simulink model "FullBalekaRaibert"  (R2025a)
settings: Solver=VariableStepAuto  StartTime=0.0  StopTime=20  RelTol=1e-3
libraries: aru_toolbox x4, simulink x2
settings Model: Creator=Gavin  LastModifiedBy=Gavin
settings ExplorerConfigSet: InternalSimMechanicsExplorerSettings=|
  | <ExplorerConfiguration>
  | 
  |   <canonicalview>default</canonicalview>
  | 
  |   <TilePanel>
  |     <TileInfo>
  |       <Tiles Columns="1" Count="1" Height="832" Rows="1" Width="1462">
  |         <Row Weight="1"/>
  |         <Column Weight="1"/>
  |         <Tile Height="1" Width="1" X="0" Y="0"/>
  |       </Tiles>
  |     </TileInfo>
  |     <SceneInfo>
  |       <SceneViewer>
  |         <IsThisViewStd>
  |           <IsStandardView>off</IsStandardView>
  |           <StandardViewName>Front</StandardViewName>
  |         </IsThisViewStd>
  |         <BGColor>
  |           <R>1</R>
  |           <G>1</G>
  |           <B>1</B>
  |           <A>1</A>
  |         </BGColor>
  |         <Camera>
  |           <DoPerspective>off</DoPerspective>
  |           <Position>
  |             <X>5.3584715991237664</X>
  |             <Y>-23.628300699422176</Y>
  |             <Z>4.8241020067654929</Z>
  |           </Position>
  |           <Center>
  |             <X>-0.00083063994179468563</X>
  |             <Y>-0.0051618537568766925</Y>
  |             <Z>0.24669244118891392</Z>
  |           </Center>
  |           <Up>
  |             <X>-0.22205533792545343</X>
  |             <Y>0.13668780175983591</Y>
  |             <Z>0.9654055478133925</Z>
  |           </Up>
  |           <XLim>2.6471256395411848</XLim>
  |           <YLim>2.6471256395411848</YLim>
  |           <ViewLimDist>0.01</ViewLimDist>
  |         </Camera>
  |       </SceneViewer>
  |     </SceneInfo>
  |   </TilePanel>
  | 
  |   <MechEditorPanel>
  |     <GfxPanelCameraMap/>
  |     <Cameras>
  |       <Camera>
  |         <Id>Camera1</Id>
  |         <Value>
  |           <Name>FollowBot</Name>
  |           <NativeCamera>
  |             <PositionTrackingFeature>Subsystem.Half_Baleka_Simscape_WIP.Planarising_Boom.Center_to_CameraUp.F</PositionTrackingFeature>
  |             <CenterTrackingFeature>Subsystem.Half_Baleka_Simscape_WIP.Planarising_Boom.Center_to_Camera.B</CenterTrackingFeature>
  |             <UpVectorTrackingFeature>Subsystem.Half_Baleka_Simscape_WIP.Planarising_Boom.Center_to_Camera.B</UpVectorTrackingFeature>
  |             <CenterTrackingOrigin>on</CenterTrackingOrigin>
  |             <UpVectorTrackingDirection>+Y</UpVectorTrackingDirection>
  |           </NativeCamera>
  |         </Value>
  |       </Camera>
  |     </Cameras>
  |     <VideoCreator>
  |       <IncludeTiles>All</IncludeTiles>
  |       <IncludeTime>on</IncludeTime>
  |       <IncludeWorldFrame>off</IncludeWorldFrame>
  |       <PlaybackSpeedRatio>1</PlaybackSpeedRatio>
  |       <FrameRate>30</FrameRate>
  |       <FrameSize>auto</FrameSize>
  |       <VideoFormat>MotionJPEGAVI</VideoFormat>
  |     </VideoCreator>
  |   </MechEditorPanel>
  | 
  |   <PlaybackSettings>
  |     <PlaybackSpeedFactor>1</PlaybackSpeedFactor>
  |   </PlaybackSettings>
  | 
  | </ExplorerConfiguration>

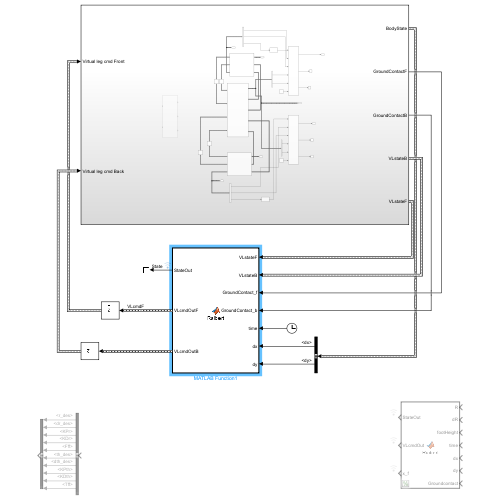
[thumbnail: Simulink's stored preview of the top-level diagram]
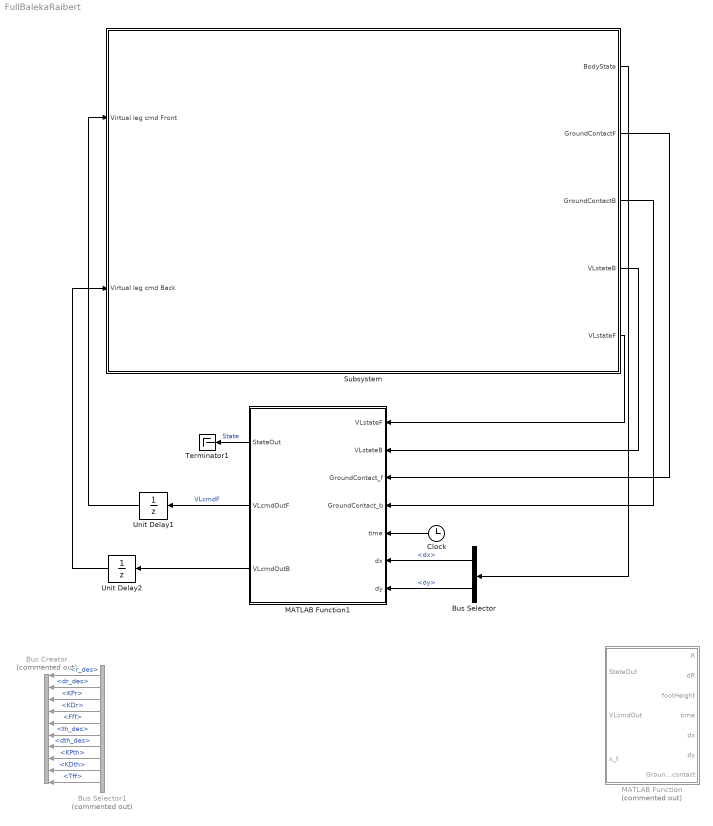
== system FullBalekaRaibert ==
  Bus Creator : BusCreator  Commented=on  Inputs=10  OutDataTypeStr=Bus: VLcmd  NonVirtualBus=on
      settings: InheritFromInputs=off
  Bus Selector : BusSelector  OutputSignals=dx,dy
  Bus Selector1 : BusSelector  Commented=on  OutputSignals=r_des,dr_des,KPr,KDr,Fff,th_des,dth_des,KPth,KDth,Tff
  Clock : Clock
  MATLAB Function : MATLAB Function  Commented=on  TreatAsAtomicUnit=on
  MATLAB Function1 : MATLAB Function  TreatAsAtomicUnit=on
  Subsystem : Subsystem
  Terminator1 : Terminator
  Unit Delay1 : UnitDelay  SampleTime=-1  HasFrameUpgradeWarning=on
  Unit Delay2 : UnitDelay  SampleTime=-1  HasFrameUpgradeWarning=on
  wires:
  MATLAB Function1/1(StateOut) -> Terminator1/1  "State"
  Clock/1 -> MATLAB Function1/5(time)
  Bus Selector/1 -> MATLAB Function1/6(dx)  "<dx>"
  Bus Selector/2 -> MATLAB Function1/7(dy)  "<dy>"
  Bus Selector1/8 -> Bus Creator/8  "<KPth>"
  Bus Selector1/2 -> Bus Creator/2  "<dr_des>"
  Bus Selector1/4 -> Bus Creator/4  "<KDr>"
  Bus Selector1/7 -> Bus Creator/7  "<dth_des>"
  Bus Selector1/5 -> Bus Creator/5  "<Fff>"
  Bus Selector1/6 -> Bus Creator/6  "<th_des>"
  Bus Selector1/3 -> Bus Creator/3  "<KPr>"
  Bus Selector1/10 -> Bus Creator/10  "<Tff>"
  Bus Selector1/9 -> Bus Creator/9  "<KDth>"
  Bus Selector1/1 -> Bus Creator/1  "<r_des>"
  MATLAB Function1/2(VLcmdOutF) -> Unit Delay1/1  "VLcmdF"
  Unit Delay1/1 -> Subsystem/1(Virtual leg cmd Front)
  MATLAB Function1/3(VLcmdOutB) -> Unit Delay2/1
  Unit Delay2/1 -> Subsystem/2(Virtual leg cmd Back)
  Subsystem/1(BodyState) -> Bus Selector/1
  Subsystem/4(VLstateB) -> MATLAB Function1/2(VLstateB)
  Subsystem/3(GroundContactB) -> MATLAB Function1/4(GroundContact_b)
  Subsystem/2(GroundContactF) -> MATLAB Function1/3(GroundContact_f)
  Subsystem/5(VLstateF) -> MATLAB Function1/1(VLstateF)

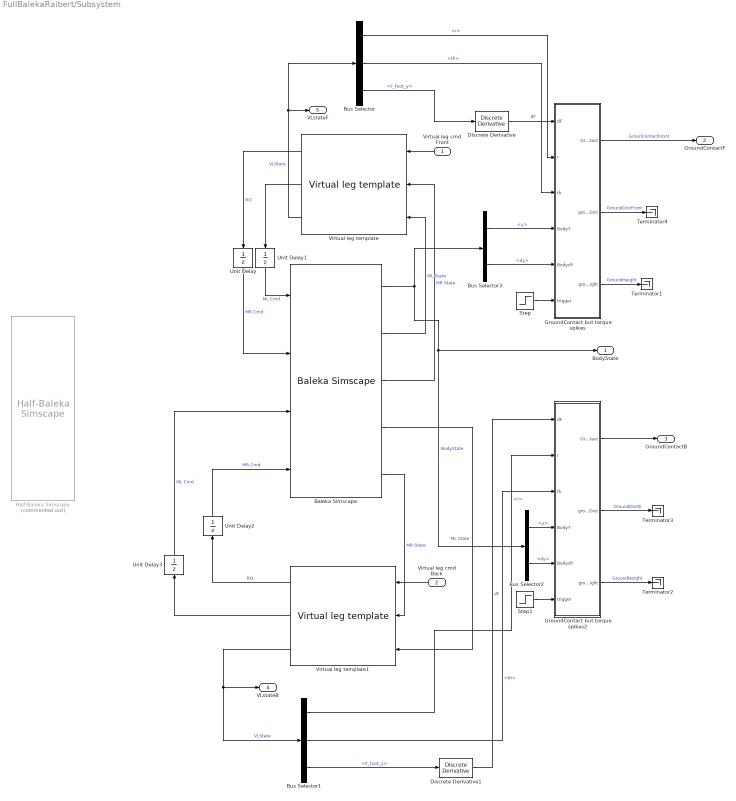
== system FullBalekaRaibert/Subsystem ==
  Virtual leg cmd Front : Inport  OutDataTypeStr=Bus: VLcmd
  Virtual leg cmd Back : Inport  Port=2  OutDataTypeStr=Bus: VLcmd
  Baleka Simscape : aru_toolbox/Baleka 2.5/Baleka Simscape  communication_rate=1000  GravityBool=on  mu_s=1  mu_k=0.9  foot_k=1e5  foot_d=1e4  y_start=0.25  StartingMode=Crouched  LOffset=3*pi/2  ROffset=-pi/2
      settings: SourceProductName=ARU Toolbox
  Bus Selector : BusSelector  OutputSignals=r,th,F_foot_y
  Bus Selector1 : BusSelector  OutputSignals=r,th,F_foot_y
  Bus Selector2 : BusSelector  OutputSignals=y,dy
  Bus Selector3 : BusSelector  OutputSignals=y,dy
  Discrete Derivative : simulink/Discrete/Discrete Derivative  gainval=1.0  ICPrevScaledInput=0.0  OutMin=[]  OutMax=[]  OutDataType=fixdt(1, 16)  OutScaling=2^-10  DoSatur=off
  Discrete Derivative1 : simulink/Discrete/Discrete Derivative  gainval=1.0  ICPrevScaledInput=0.0  OutMin=[]  OutMax=[]  OutDataType=fixdt(1, 16)  OutScaling=2^-10  DoSatur=off
  GroundContact but torque spikes : MATLAB Function  TreatAsAtomicUnit=on
  GroundContact but torque spikes2 : MATLAB Function  TreatAsAtomicUnit=on
  Half-Baleka Simscape : aru_toolbox/Baleka 2.5/Half-Baleka Simscape  Commented=on  communication_rate=1000  GravityBool=on  mu_s=1  mu_k=0.9  foot_k=1e5  foot_d=1e4  y_start=0.3  StartingMode=Zero (set Starting values manually)  LOffset=4.1  ROffset=-0.88
      settings: SourceProductName=ARU Toolbox
  Step : Step  Time=0.005  SampleTime=0
  Step1 : Step  Time=0.005  SampleTime=0
  Terminator{1..4} (4 alike) : Terminator
  Unit Delay{,1..3} (4 alike) : UnitDelay  SampleTime=-1  HasFrameUpgradeWarning=on
  Virtual leg template : aru_toolbox/Baleka 2.5/Virtual leg template  mx_tune=1  cx_tune=0  my_tune=1  cy_tune=0
      settings: SourceProductName=ARU Toolbox
  Virtual leg template1 : aru_toolbox/Baleka 2.5/Virtual leg template  mx_tune=1  cx_tune=0  my_tune=1  cy_tune=0
      settings: SourceProductName=ARU Toolbox
  BodyState : Outport
  GroundContactF : Outport  Port=2
  GroundContactB : Outport  Port=3
  VLstateB : Outport  Port=4
  VLstateF : Outport  Port=5
  wires:
  Bus Selector/1 -> GroundContact but torque spikes/2(r)  "<r>"
  Unit Delay1/1 -> Baleka Simscape/1  "ML Cmd"
  Virtual leg cmd Front/1 -> Virtual leg template/1
  Virtual leg template/3 -> Bus Selector/1, VLstateF/1  "VLState"
  Baleka Simscape/3 -> Virtual leg template/2  "MR State"
  Baleka Simscape/2 -> Virtual leg template/3  "ML State"
  Virtual leg template/1 -> Unit Delay/1  "RO"
  Bus Selector/2 -> GroundContact but torque spikes/3(th)  "<th>"
  Unit Delay/1 -> Baleka Simscape/2  "MR Cmd"
  Bus Selector/3 -> Discrete Derivative/1  "<F_foot_y>"
  GroundContact but torque spikes/1(GroundContact) -> GroundContactF/1  "GrounContactFront"
  Virtual leg template/2 -> Unit Delay1/1
  Bus Selector3/1 -> GroundContact but torque spikes/4(BodyY)  "<y>"
  Bus Selector3/2 -> GroundContact but torque spikes/5(BodydY)  "<dy>"
  GroundContact but torque spikes/3(groundHeight) -> Terminator1/1  "GroundHeight"
  Discrete Derivative/1 -> GroundContact but torque spikes/1(dF)  "dF"
  GroundContact but torque spikes/2(groundDist) -> Terminator4/1  "GroundDistFront"
  Step/1 -> GroundContact but torque spikes/6(trigger)
  Baleka Simscape/4 -> Virtual leg template1/3  "ML State"
  Unit Delay2/1 -> Baleka Simscape/4  "MR Cmd"
  Virtual leg cmd Back/1 -> Virtual leg template1/1
  Baleka Simscape/1 -> Bus Selector2/1, BodyState/1, Bus Selector3/1  "BodyState"
  Bus Selector2/2 -> GroundContact but torque spikes2/5(BodydY)  "<dy>"
  GroundContact but torque spikes2/2(groundDist) -> Terminator3/1  "GroundDistB"
  Unit Delay3/1 -> Baleka Simscape/3  "ML Cmd"
  Bus Selector1/1 -> GroundContact but torque spikes2/2(r)  "<r>"
  Virtual leg template1/1 -> Unit Delay2/1  "RO"
  Virtual leg template1/3 -> VLstateB/1, Bus Selector1/1  "VLState"
  Baleka Simscape/5 -> Virtual leg template1/2  "MR State"
  Bus Selector1/3 -> Discrete Derivative1/1  "<F_foot_y>"
  GroundContact but torque spikes2/1(GroundContact) -> GroundContactB/1
  GroundContact but torque spikes2/3(groundHeight) -> Terminator2/1  "GroundHeight"
  Virtual leg template1/2 -> Unit Delay3/1
  Bus Selector2/1 -> GroundContact but torque spikes2/4(BodyY)  "<y>"
  Bus Selector1/2 -> GroundContact but torque spikes2/3(th)  "<th>"
  Step1/1 -> GroundContact but torque spikes2/6(trigger)
  Discrete Derivative1/1 -> GroundContact but torque spikes2/1(dF)  "dF"

== matlab function FullBalekaRaibert/MATLAB Function ==
  settings: updateMethod=DISCRETE  sampleTime=0.001
  data: R input; StateOut output; dR input; footHeight input; time input; dx input; dy input; VLcmdOut output Bus: VLcmd; Groundcontact input; x_f output
function [StateOut, VLcmdOut, x_f]   = Raibert(R, dR,footHeight, time,dx, dy, Groundcontact)
    % Raibert hopping state machine
    persistent state landTime VLcmd x_f_des %dR
    % State variable
    % 0 = SETUP
    % 1 = FLIGHT
    % 2 = COMPRESSION
    % 3 = THRUST
    
    % Params:
    Ts = 0.25;
    Kdx = -0.01;
    dx_d = 2;


    x_f = dx*Ts/2 + Kdx*(dx - dx_d); % Foot placement
    % x_f = 0.1;
    
    if isempty(state)
        state = 0;
        x_f_des = 0;
        landTime = 99;
        % dR = 0;
        VLcmd.r_des = 0.45;
        VLcmd.dr_des =0;
        VLcmd.KPr = 1000;
        VLcmd.KDr =40;
        VLcmd.Fff =0;
        VLcmd.th_des = -pi/2;
        VLcmd.dth_des =0;
        VLcmd.KPth = 200;
        VLcmd.KDth = 20;
        VLcmd.Tff = 0;
        
    end

switch state
    case 0 % SETUP
        % Specific commands for first landing
        VLcmd.r_des = 0.25;
        VLcmd.dr_des =0;
        VLcmd.KPr = 600;
        VLcmd.KDr =20;
        VLcmd.Fff =0;

        VLcmd.th_des = -pi/2 + asin(-0.07/R);
        VLcmd.KPth = 200;
        VLcmd.KDth = 20;
        % if Groundcontact % On foot touching ground go to COMPRESSION
        if time >0.5 % wait for setup
            state = 4;
            landTime = time;
            x_f_des = 0.07;

        end
    case 1 % FLIGHT
        % Brace for impact with high-ish spring
        VLcmd.r_des = 0.45;
        VLcmd.dr_des =0;
        VLcmd.KPr = 600;
        VLcmd.KDr =20;
        VLcmd.Fff = 0;
        % Position leg for landing
        VLcmd.th_des = -pi/2 + asin(x_f/R);
        VLcmd.dth_des = 0;
        VLcmd.KPth = 600;
        VLcmd.KDth = 20;

        if Groundcontact % On foot touching ground go to COMPRESSION
            state = 2;
            landTime = time;
            x_f_des = x_f;
        end
    case 2 % COMPRESSION
        % Let spring compress
        VLcmd.r_des = 0.45;
        VLcmd.dr_des =0;
        VLcmd.KPr = 900;
        VLcmd.KDr =10;
        VLcmd.Fff = 0;
        % Servo hip
        VLcmd.th_des = -pi/2- asin(x_f_des/R); 
        VLcmd.dth_des = 0;%(dx*R - dR*R*sin(th))/(cos(th)*R^2);
        VLcmd.KPth = 800;
        VLcmd.KDth = 50;
        % When leg stops compressing (dR = 0) go to THRUST
        if (((time-landTime)>0.05)&&(dR>0)) 
            state = 3;
        end
    case 3 % THRUST
        % Apply upwards thrust force
        VLcmd.r_des = 0.6;
        VLcmd.dr_des =0;
        VLcmd.KPr = 5000;
        VLcmd.KDr =0;
        VLcmd.Fff = 0;% 2000;

        % Servo hip
        VLcmd.th_des = -pi/2 - asin(x_f_des/R); 
        VLcmd.dth_des = 0;%(dx*R - dR*R*sin(th))/(cos(th)*R^2);
        VLcmd.KPth = 800;
        VLcmd.KDth = 50;

        if ~Groundcontact%&&(dy>0))% ||((th1>3*pi/2)||(th2<-pi/2))
            state =1;
        end
    case 4 % StartingTHRUST
        % Apply upwards thrust force
        VLcmd.r_des = 0.6;
        VLcmd.dr_des =0;
        VLcmd.KPr = 1500;
        VLcmd.KDr =0;
        VLcmd.Fff = 0;% 2000;

        % Servo hip
        VLcmd.th_des = -pi/2 - asin(x_f_des/R); 
        VLcmd.dth_des = 0;%(dx*R - dR*R*sin(th))/(cos(th)*R^2);
        VLcmd.KPth = 800;
        VLcmd.KDth = 75;

        if ~Groundcontact%&&(dy>0))% ||((th1>3*pi/2)||(th2<-pi/2))
            state =1;
        end

end
    VLcmdOut.r_des = VLcmd.r_des;
    VLcmdOut.dr_des = VLcmd.dr_des;
    VLcmdOut.KPr = VLcmd.KPr;
    VLcmdOut.KDr = VLcmd.KDr;
    VLcmdOut.Fff = VLcmd.Fff;

    VLcmdOut.th_des = VLcmd.th_des;
    VLcmdOut.dth_des = VLcmd.dth_des;
    VLcmdOut.KPth = VLcmd.KPth;
    VLcmdOut.KDth = VLcmd.KDth;
    VLcmdOut.Tff = VLcmd.Tff;

    StateOut = state;
end

== matlab function FullBalekaRaibert/Subsystem/GroundContact but torque spikes ==
  settings: updateMethod=DISCRETE  sampleTime=0.001
  data: dF input; r input; th input; GroundContact output; BodyY input; groundDist output; groundHeight output; BodydY input; trigger input
function [GroundContact, groundDist, groundHeight]  = ImpactTorque(dF,r, th, BodyY, BodydY, trigger)
        % need to see how IRL torque spikes work, but we can do a veeery
        % rough guestimate here:
        persistent GroundContactpers;
        persistent GroundHeight;
        if isempty(GroundContactpers)
            GroundContactpers = true;
            GroundHeight = 0;
        end
        if trigger >0
        %     GroundContactpers = true;
        %     GroundHeight = BodyY  +sin(th)*r;
        % end
        groundDist = BodyY + sin(th)*r;% - 0.004
            if ~GroundContactpers % Impact sensing for gnd
               if (dF<-3e4) && (BodydY <0) && (groundDist <0.1)
                GroundContactpers = true;
                GroundHeight = BodyY  +sin(th)*r; % - 0.004
               end
               groundDist=BodyY + sin(th)*r;
            else 
                % leg length calc for flight
                
                if BodydY >0
                    GroundContactpers = ~(groundDist>0.005+GroundHeight);
                end
            end

        else
            groundDist=BodyY + sin(th)*r;
        end
          
        GroundContact = GroundContactpers;
        groundHeight = GroundHeight;
end

== matlab function FullBalekaRaibert/MATLAB Function1 ==
  settings: updateMethod=DISCRETE  sampleTime=0.001
  data: VLstateF input Bus: VLState; StateOut output; VLstateB input Bus: VLState; GroundContact_f input; GroundContact_b input; time input; dx input; dy input; VLcmdOutF output Bus: VLcmd; VLcmdOutB output Bus: VLcmd
function [StateOut, VLcmdOutF, VLcmdOutB] = Raibert(VLstateF, VLstateB, GroundContact_f, GroundContact_b, time, dx, dy)
    % Raibert hopping state machine
    persistent state landTime VLcmd_f VLcmd_b x_f_des
    % State variable
    % 0 = SETUP
    % 1 = FLIGHT (front)
    % 2 = COMPRESSION (front)
    % 3 = THRUST (front)
    % 4 = FLIGHT (back)
    % 5 = COMPRESSION (back)
    % 6 = THRUST (back)
    
    % Params:
    Ts = 0.12;
    Kdx = -0.05;
    % Kdx = 0.1;
    dx_d = 2;

    FloatLeg = 0.22;
    GroundLeg = 0.40;

    
     

    x_f = dx*Ts/2 + Kdx*(dx - dx_d); % Foot placement
    % x_f = 0.1;

    % dR_f = cmd_f(5);
    % dR_b = cmd_b(5);
    % [R_f, th] = BalekaKinematicsRth(th1, th2);
    % [R_b, th] = BalekaKinematicsRth(th3, th4);
    R_f = VLstateF.r;
    R_b = VLstateB.r;

    dR_f = VLstateF.dr;
    dR_b = VLstateB.dr;


    %% Set up reused constants for simple editing

    % Landing
    VL_landing.r_des = GroundLeg;
    VL_landing.KPr = 1000;
    VL_landing.KDr =40;
    VL_landing.KPth = 200;
    VL_landing.KDth = 20;

    VL_landing.dr_des = 0;
    VL_landing.dth_des = 0;
    VL_landing.Fff = 0;
    VL_landing.Tff = 0;
    VL_landing.th_des = 0;
    
    
    % Floating

    VL_float.r_des = FloatLeg;
    VL_float.KPr = 1000;
    VL_float.KDr =40;
    VL_float.KPth = 200;
    VL_float.KDth = 20;

  
    VL_float.dr_des = 0;
    VL_float.dth_des = 0;
    VL_float.Fff = 0;
    VL_float.Tff = 0;
    VL_float.th_des = 0;

    % Compress
    VL_compress.r_des = GroundLeg;
    VL_compress.KPr = 1500;
    VL_compress.KDr =50;
    VL_compress.KPth = 600;
    VL_compress.KDth = 20;

    VL_compress.dr_des = 0;
    VL_compress.dth_des = 0;
    VL_compress.Fff =0;
    VL_compress.Tff = 0;
    VL_compress.th_des = 0;

    % Thrust

    VL_thrust.r_des = 0.6;
    VL_thrust.KPr = 7000;
    VL_thrust.KDr =0;
    VL_thrust.KPth = 800;
    VL_thrust.KDth = 50;

    VL_thrust.dr_des = 0;
    VL_thrust.dth_des = 0;
    VL_thrust.Fff =0;
    VL_thrust.Tff = 0;
    VL_thrust.th_des = 0;


    if isempty(state)
        state = 0;
        landTime = 99;
        dR_f = 0;
        dR_b = 0;
        x_f_des = 0;
        VLcmd_f = VL_compress;
        VLcmd_f.th_des = -pi/2;
        VLcmd_b = VL_compress;
        VLcmd_b.th_des = -pi/2;
    end

switch state
    case 0 % SETUP
        % Specific commands for first landing
        VLcmd_f = VL_landing;
        VLcmd_f.r_des = 0.25;
        VLcmd_f.th_des = -pi/2 +asin(-0.07/R_f);
        
        VLcmd_b = VL_landing;
        VLcmd_b.r_des = 0.25;
        VLcmd_b.th_des = -pi/2 +asin(-0.07/R_f);

        % VLcmd_b = VL_float;
        % VLcmd_b.th_des = -pi/2;
        % 
        % if (footHeight_f <=0)&&(dy<0) % On foot touching ground go to COMPRESSION
        if time >0.5
            state = 2;
            landTime = time;
            x_f_des = 0.07;

        end
    case 1 % FLIGHT (front)
        % Brace for impact with high-ish spring
        VLcmd_f = VL_landing;
        VLcmd_f.th_des = -pi/2 +asin(x_f/R_f);

        VLcmd_b = VL_float;
        VLcmd_b.th_des = -pi/2;% + asin(x_f_des/R_b);


        if GroundContact_f % On foot touching ground go to COMPRESSION
            state = 2;
            landTime = time;
            x_f_des = x_f;
        end
    case 2 % COMPRESSION (front)
        % Let spring compress
        VLcmd_f = VL_compress;
        VLcmd_f.th_des = -pi/2- asin(x_f_des/R_f); 

        VLcmd_b = VL_float;
        VLcmd_b.th_des = -pi/2;% + asin(x_f_des/R_b);

        % When leg stops compressing (dR = 0) go to THRUST
        if (((time-landTime)>0.05)&&(dR_f>0)) 
            state = 3;
        end
    case 3 % THRUST (front)
        % Apply upwards thrust force
        VLcmd_f = VL_thrust;
        VLcmd_f.th_des = -pi/2 - asin(x_f_des/R_f);

        VLcmd_b = VL_float;
        VLcmd_b.th_des = -pi/2;% + asin(x_f_des/R_b);

        if ~GroundContact_f%&&(dy>0))% ||((th1>3*pi/2)||(th2<-pi/2))
            state =4;
        end

    case 4 % FLIGHT (back)
        VLcmd_f = VL_float;
        VLcmd_f.th_des = -pi/2;% + asin(x_f_des/R_f);

        VLcmd_b = VL_landing;
        VLcmd_b.th_des = -pi/2 + asin(x_f/R_b);

        if GroundContact_b % On foot touching ground go to COMPRESSION
            state = 5;
            landTime = time;
            x_f_des = x_f;
        end
    case 5 % COMPRESSION (back)
        VLcmd_f = VL_float;
        VLcmd_f.th_des = -pi/2;% + asin(x_f_des/R_f);
        VLcmd_f.KPr = 4000;

        VLcmd_b = VL_compress;
        VLcmd_b.th_des = -pi/2- asin(x_f_des/R_b); 
        VLcmd_b.KPr = 4000;

        % When leg stops compressing (dR = 0) go to THRUST
        if (((time-landTime)>0.05)&&(dR_b>0)) 
            state = 6;
        end
    case 6 % THRUST (back)
        % Apply upwards thrust force
        VLcmd_f = VL_float;
        VLcmd_f.th_des = -pi/2;% + asin(x_f_des/R_f);

        VLcmd_b = VL_thrust;
        VLcmd_b.th_des = -pi/2 - asin(x_f_des/R_b);

        if ~GroundContact_b %&&(dy>0))% ||((th1>3*pi/2)||(th2<-pi/2))
            state =1;
        end
    case 7 % THRUST (BOTH)
        % Apply upwards thrust force
        VLcmd_f = VL_thrust;
        VLcmd_f.th_des = -pi/2 - asin(x_f_des/R_f);

        VLcmd_b = VL_thrust;
        VLcmd_b.th_des = -pi/2 - asin(x_f_des/R_b);

        if ~GroundContact_b%&&(dy>0))% ||((th1>3*pi/2)||(th2<-pi/2))
            state =1;
        end

end
    VLcmdOutF.r_des = VLcmd_f.r_des;
    VLcmdOutF.dr_des = VLcmd_f.dr_des;
    VLcmdOutF.KPr = VLcmd_f.KPr;
    VLcmdOutF.KDr = VLcmd_f.KDr;
    VLcmdOutF.Fff = VLcmd_f.Fff;

    VLcmdOutF.th_des = VLcmd_f.th_des;
    VLcmdOutF.dth_des = VLcmd_f.dth_des;
    VLcmdOutF.KPth = VLcmd_f.KPth;
    VLcmdOutF.KDth = VLcmd_f.KDth;
    VLcmdOutF.Tff = VLcmd_f.Tff;

    VLcmdOutB.r_des = VLcmd_b.r_des;
    VLcmdOutB.dr_des = VLcmd_b.dr_des;
    VLcmdOutB.KPr = VLcmd_b.KPr;
    VLcmdOutB.KDr = VLcmd_b.KDr;
    VLcmdOutB.Fff = VLcmd_b.Fff;

    VLcmdOutB.th_des = VLcmd_b.th_des;
    VLcmdOutB.dth_des = VLcmd_b.dth_des;
    VLcmdOutB.KPth = VLcmd_b.KPth;
    VLcmdOutB.KDth = VLcmd_b.KDth;
    VLcmdOutB.Tff = VLcmd_b.Tff;
    
    StateOut = state;
end

== matlab function FullBalekaRaibert/Subsystem/GroundContact but torque spikes2 ==
  settings: updateMethod=DISCRETE  sampleTime=0.001
  data: dF input; r input; th input; GroundContact output; BodyY input; groundDist output; groundHeight output; BodydY input; trigger input
function [GroundContact, groundDist, groundHeight]  = ImpactTorque(dF,r, th, BodyY, BodydY, trigger)
        % need to see how IRL torque spikes work, but we can do a veeery
        % rough guestimate here:
        persistent GroundContactpers;
        persistent GroundHeight;
        if isempty(GroundContactpers)
            GroundContactpers = true;
            GroundHeight = 0;
        end
        if trigger >0
        %     GroundContactpers = true;
        %     GroundHeight = BodyY  +sin(th)*r;
        % end
        groundDist = BodyY + sin(th)*r;% - 0.004
            if ~GroundContactpers % Impact sensing for gnd
               if (dF<-3e4) && (BodydY <0) && (groundDist <0.1)
                GroundContactpers = true;
                GroundHeight = BodyY  +sin(th)*r; % - 0.004
               end
               groundDist=BodyY + sin(th)*r;
            else 
                % leg length calc for flight
                
                if BodydY >0
                    GroundContactpers = ~(groundDist>0.005+GroundHeight);
                end
            end

        else
            groundDist=BodyY + sin(th)*r;
        end
          
        GroundContact = GroundContactpers;
        groundHeight = GroundHeight;
end
